simulink model "step_transient"  (R2023b)
settings: Solver=FixedStepDiscrete  StartTime=0.0  StopTime=inf  FixedStep=1e-4  RelTol=1e-3
libraries: speedgoatlib_IO102 x2
settings Model: Creator=wasynczu  LastModifiedBy=mluser
settings SolverCC: ConcurrentTasks=on  PositivePriorityOrder=on
settings OptimizationCC: BlockReduction=off  OptimizeBlockIOStorage=off
settings DebuggingCC: TasksWithSamePriorityMsg=none  UnconnectedInputMsg=warning  UnconnectedOutputMsg=warning  UnconnectedLineMsg=warning
settings HardwareCC: ProdBitPerLong=64  ProdLongLongMode=on  ProdHWDeviceType=Intel->x86-64 (Linux 64)
settings ModelReferenceCC: EnableRefExpFcnMdlSchedulingChecks=on
settings RTWCC: Description=Simulink Real-Time  SystemTargetFile=slrealtime.tlc  TemplateMakefile=slrealtime_default_tmf  Toolchain=Simulink Real-Time Toolchain  BuildConfiguration=Faster Runs  CodeExecutionProfiling=on  TargetLang=C++  DLArmComputeVersion=19.05

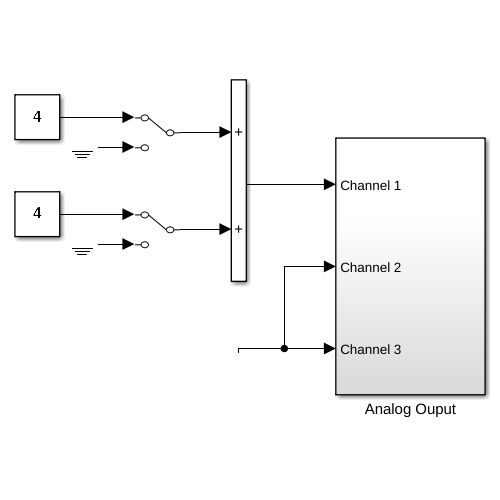
[thumbnail: Simulink's stored preview of the top-level diagram]
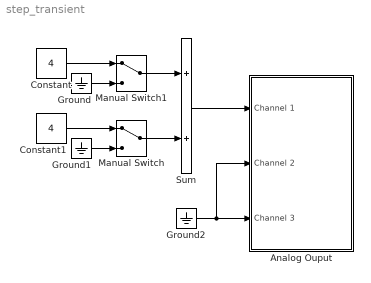
== system step_transient ==
  Analog Ouput : Subsystem
  Constant : Constant  Value=4
  Constant1 : Constant  Value=4
  Ground : Ground
  Ground1 : Ground
  Ground2 : Ground
  Manual Switch : ManualSwitch
  Manual Switch1 : ManualSwitch
  Sum : Sum
  wires:
  Sum/1 -> Analog Ouput/1(Channel 1)
  Manual Switch1/1 -> Sum/1
  Manual Switch/1 -> Sum/2
  Ground/1 -> Manual Switch1/2
  Ground2/1 -> Analog Ouput/2(Channel 2), Analog Ouput/3(Channel 3)
  Ground1/1 -> Manual Switch/2
  Constant/1 -> Manual Switch1/1
  Constant1/1 -> Manual Switch/1

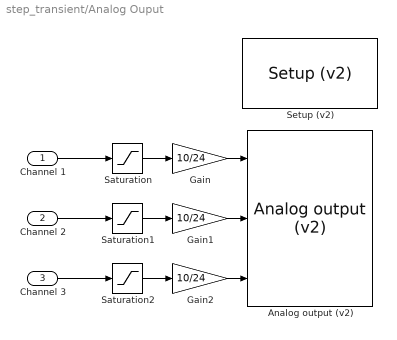
== system step_transient/Analog Ouput ==
  Channel 1 : Inport
  Channel 2 : Inport  Port=2
  Channel 3 : Inport  Port=3
  "Analog output (v2) " : speedgoatlib_IO102/Analog output (v2)   id=1  channels=[1 2 3]  range=1  ts=-1  pciSlot=-1
  Gain : Gain  Gain=10/24
  Gain1 : Gain  Gain=10/24
  Gain2 : Gain  Gain=10/24
  Saturation : Saturate  UpperLimit=24  LowerLimit=-24
  Saturation1 : Saturate  UpperLimit=24  LowerLimit=-24
  Saturation2 : Saturate  UpperLimit=24  LowerLimit=-24
  "Setup (v2) " : speedgoatlib_IO102/Setup (v2)   id=1  range=+-10V  cal=off  pciSlot=-1  adCoupling=Single-ended  adChannelMode=Multiple-channel (enter number of channels below)  adChannel=4  daChannel=[1,2,3]  daInitValue=[0]  daReset=[1]  DioDirectionLo=Input  DioDirectionHi=Output  doChannel=[9]  doInitValue=[0]  doReset=[1]  diChannel=[1]
  wires:
  Channel 1/1 -> Saturation/1
  Channel 3/1 -> Saturation2/1
  Channel 2/1 -> Saturation1/1
  Gain2/1 -> "Analog output (v2) "/3
  Gain/1 -> "Analog output (v2) "/1
  Gain1/1 -> "Analog output (v2) "/2
  Saturation2/1 -> Gain2/1
  Saturation1/1 -> Gain1/1
  Saturation/1 -> Gain/1
